simulink model "GTA_PCMFirmware"  (Simulink 7.8)
settings: Solver=FixedStepDiscrete  StartTime=0.0  StopTime=10.0  RelTol=1e-3
PreLoadFcn:
  | try, eval([bdroot '_setup']); catch, eval('model_setup', ''); end
InitFcn:
  | try, eval([bdroot '_setup']); catch, eval('model_setup', ''); end
undefined symbols (not defined in the file): fndFwd, fndNeut, fndRev, FWDlockout, GCM, keySwIgn2, motohawk_build_version, motohawk_trunc_name, motohawk_vardec_path, REVlockout
libraries: MotoHawk_lib x313, simulink x47, GTA_Library x13
(part 2 of 7)

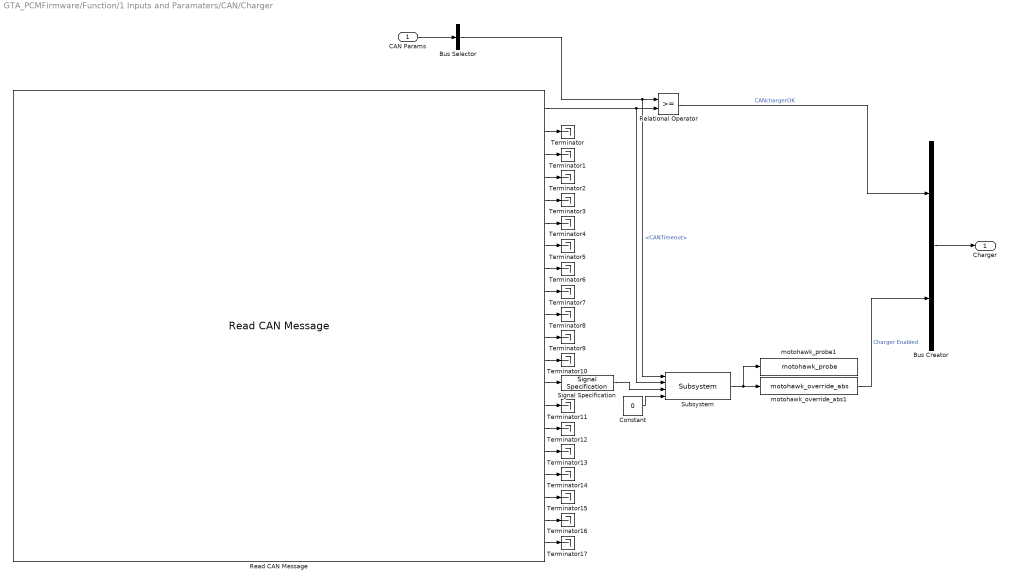
== system GTA_PCMFirmware/Function/1 Inputs and Paramaters/CAN/Charger ==
  CAN Params : Inport
  Bus Creator : BusCreator  Inputs=2
  Bus Selector : BusSelector  OutputSignals=CANTimeout
  Constant : Constant  Value=0  OutDataTypeStr=boolean
  Read CAN Message : MotoHawk_lib/CAN Blocks/Read CAN Message  nam='BMS_CAN'  bus=-2  msg=CANMSG_LHVcharger_Status  queue=1  slot=''  valid=off  stale=on  labelwires=off
  Relational Operator : RelationalOperator  OutDataTypeStr=boolean
  Signal Specification : SignalSpecification  OutDataTypeStr=boolean
  Subsystem : GTA_Library/Subsystem
  Terminator{,1..17} (18 alike) : Terminator
  motohawk_override_abs1 : MotoHawk_lib/Calibration & Probing Blocks/motohawk_override_abs  parent_name='ChargerEnabled'  parent_val=0  show_more=off  name_source=Use Parameter  parent_read_level=1  parent_override_level=1  view_as=Number  enum_struct={'Disabled', 'Enabled'}  use_help_units=off  parent_help=''  parent_units=''  use_min_max=off  parent_min=-inf  parent_max=inf  use_precision=off  parent_precision=''  parent_gain=1  parent_offset=0  parent_exp=1  use_mototune_group=off  parent_group=motohawk_vardec_path(gcb)
  motohawk_probe1 : MotoHawk_lib/Calibration & Probing Blocks/motohawk_probe  nam='ChargerEnabled'  show_more=off  name_source=Use Parameter  read_level=1  view_as=Number  enum_struct={'Disabled', 'Enabled'}  vector_style=Wide Row  use_help_units=off  help=''  units=''  use_header_enum=off  row_header_enum={}  col_header_enum={}  use_min_max=off  min_val=-inf  max_val=inf  use_precision=off  precision=''  gain=1  offset=0  exp=1  use_mototune_group=off  mototune_group=motohawk_vardec_path(gcb)
  Charger : Outport
  wires:
  CAN Params/1 -> Bus Selector/1
  Bus Selector/1 -> Relational Operator/1, Subsystem/1  "<CANTimeout>"
  Read CAN Message/1 -> Relational Operator/2, Subsystem/2
  Read CAN Message/2 -> Terminator/1
  Read CAN Message/3 -> Terminator1/1
  Read CAN Message/4 -> Terminator2/1
  Read CAN Message/5 -> Terminator3/1
  Read CAN Message/6 -> Terminator4/1
  Read CAN Message/7 -> Terminator5/1
  Read CAN Message/8 -> Terminator6/1
  Read CAN Message/9 -> Terminator7/1
  Read CAN Message/10 -> Terminator8/1
  Read CAN Message/11 -> Terminator9/1
  Read CAN Message/12 -> Terminator10/1
  Read CAN Message/14 -> Terminator11/1
  Read CAN Message/15 -> Terminator12/1
  Read CAN Message/16 -> Terminator13/1
  Read CAN Message/17 -> Terminator14/1
  Read CAN Message/18 -> Terminator15/1
  Read CAN Message/19 -> Terminator16/1
  Read CAN Message/20 -> Terminator17/1
  Read CAN Message/13 -> Signal Specification/1
  Constant/1 -> Subsystem/4
  Signal Specification/1 -> Subsystem/3
  Relational Operator/1 -> Bus Creator/1  "CANchargerOK"
  Bus Creator/1 -> Charger/1
  Subsystem/1 -> motohawk_override_abs1/1, motohawk_probe1/1
  motohawk_override_abs1/1 -> Bus Creator/2  "Charger Enabled"

== system GTA_PCMFirmware/Function/1 Inputs and Paramaters/Digital/Brake Switch ==
  Bus Creator : BusCreator  Inputs=1
  Data Type Conversion : DataTypeConversion  OutDataTypeStr=boolean
  Relay : Relay  OnSwitchValue=500  OffSwitchValue=400  OutDataTypeStr=uint8
  motohawk_ain : MotoHawk_lib/Analog I//O Blocks/motohawk_ain  res_name='BrakeSwitch'  text_resource=AN3M  code_resource=NONE  val_resource=-1  target=GCM-0563-048-0802  resource_enum_str=(None)=-1,LSD1=25,LSD2=26,ECUP=53,DRVP=54,XDRP=55,AN1M=56,AN2M=57,AN3M=58,AN4M=59,AN5M=60,AN6M=61,AN7M=62,AN8M=63,AN9M=64,AN10M=65,AN11M=66,AN12M=67,AN13M=68,AN14M=69,AN15M=70,AN16M=71,ESTOP=97,PWMADC=142  altref=5V Reference  typ=uint16  num_adc_bits=10  use_stat=off  use_vardec=off  nam='RTD1_MW'  read_level=1  write_level=1  group='System | I/O Pins | Inputs Config'
  motohawk_override_abs : MotoHawk_lib/Calibration & Probing Blocks/motohawk_override_abs  parent_name='BrakeSwitch'  parent_val=0  show_more=off  name_source=Use Parameter  parent_read_level=1  parent_override_level=1  view_as=Number  enum_struct={'Disabled', 'Enabled'}  use_help_units=off  parent_help=''  parent_units=''  use_min_max=off  parent_min=-inf  parent_max=inf  use_precision=off  parent_precision=''  parent_gain=1  parent_offset=0  parent_exp=1  use_mototune_group=off  parent_group=motohawk_vardec_path(gcb)
  motohawk_probe : MotoHawk_lib/Calibration & Probing Blocks/motohawk_probe  nam='BrakeSwitch'  show_more=off  name_source=Use Parameter  read_level=1  view_as=Number  enum_struct={'Disabled', 'Enabled'}  vector_style=Wide Row  use_help_units=off  help=''  units=''  use_header_enum=off  row_header_enum={}  col_header_enum={}  use_min_max=off  min_val=-inf  max_val=inf  use_precision=off  precision=''  gain=1  offset=0  exp=1  use_mototune_group=off  mototune_group=motohawk_vardec_path(gcb)
  BrakeSwitch : Outport
  wires:
  motohawk_ain/1 -> Relay/1
  Relay/1 -> Data Type Conversion/1
  Data Type Conversion/1 -> motohawk_override_abs/1, motohawk_probe/1
  motohawk_override_abs/1 -> Bus Creator/1  "BrakeSw"
  Bus Creator/1 -> BrakeSwitch/1

== system GTA_PCMFirmware/Function/1 Inputs and Paramaters/Digital/Charger ==
  Bus Creator : BusCreator  Inputs=1
  Data Type Conversion : DataTypeConversion  OutDataTypeStr=boolean
  Relay : Relay  OnSwitchValue=150  OffSwitchValue=100  OutDataTypeStr=uint8
  motohawk_ain : MotoHawk_lib/Analog I//O Blocks/motohawk_ain  res_name='ACPresent'  text_resource=AN13M  code_resource=NONE  val_resource=-1  target=GCM-0563-048-0802  resource_enum_str=(None)=-1,LSD1=25,LSD2=26,ECUP=53,DRVP=54,XDRP=55,AN1M=56,AN2M=57,AN3M=58,AN4M=59,AN5M=60,AN6M=61,AN7M=62,AN8M=63,AN9M=64,AN10M=65,AN11M=66,AN12M=67,AN13M=68,AN14M=69,AN15M=70,AN16M=71,ESTOP=97,PWMADC=142  altref=5V Reference  typ=uint16  num_adc_bits=10  use_stat=off  use_vardec=off  nam='RTD1_MW'  read_level=1  write_level=1  group='System | I/O Pins | Inputs Config'
  motohawk_override_abs : MotoHawk_lib/Calibration & Probing Blocks/motohawk_override_abs  parent_name='AC_Present'  parent_val=0  show_more=off  name_source=Use Parameter  parent_read_level=1  parent_override_level=1  view_as=Number  enum_struct={'Disabled', 'Enabled'}  use_help_units=off  parent_help=''  parent_units=''  use_min_max=off  parent_min=-inf  parent_max=inf  use_precision=off  parent_precision=''  parent_gain=1  parent_offset=0  parent_exp=1  use_mototune_group=off  parent_group=motohawk_vardec_path(gcb)
  motohawk_probe : MotoHawk_lib/Calibration & Probing Blocks/motohawk_probe  nam='AC_Present'  show_more=off  name_source=Use Parameter  read_level=1  view_as=Number  enum_struct={'Disabled', 'Enabled'}  vector_style=Wide Row  use_help_units=off  help=''  units=''  use_header_enum=off  row_header_enum={}  col_header_enum={}  use_min_max=off  min_val=-inf  max_val=inf  use_precision=off  precision=''  gain=1  offset=0  exp=1  use_mototune_group=off  mototune_group=motohawk_vardec_path(gcb)
  Charger : Outport
  wires:
  motohawk_ain/1 -> Relay/1
  Relay/1 -> Data Type Conversion/1
  Bus Creator/1 -> Charger/1
  Data Type Conversion/1 -> motohawk_override_abs/1, motohawk_probe/1
  motohawk_override_abs/1 -> Bus Creator/1  "acPresent"

== system GTA_PCMFirmware/Function/1 Inputs and Paramaters/Digital/EStop ==
  Bus Creator : BusCreator  Inputs=1
  Data Type Conversion : DataTypeConversion  OutDataTypeStr=boolean
  Relay : Relay  OnSwitchValue=500  OffSwitchValue=400  OutDataTypeStr=uint8
  motohawk_ain : MotoHawk_lib/Analog I//O Blocks/motohawk_ain  res_name='EStopSwitch'  text_resource=AN12M  code_resource=NONE  val_resource=-1  target=GCM-0563-048-0802  resource_enum_str=(None)=-1,LSD1=25,LSD2=26,ECUP=53,DRVP=54,XDRP=55,AN1M=56,AN2M=57,AN3M=58,AN4M=59,AN5M=60,AN6M=61,AN7M=62,AN8M=63,AN9M=64,AN10M=65,AN11M=66,AN12M=67,AN13M=68,AN14M=69,AN15M=70,AN16M=71,ESTOP=97,PWMADC=142  altref=5V Reference  typ=uint16  num_adc_bits=10  use_stat=off  use_vardec=off  nam='RTD1_MW'  read_level=1  write_level=1  group='System | I/O Pins | Inputs Config'
  motohawk_override_abs : MotoHawk_lib/Calibration & Probing Blocks/motohawk_override_abs  parent_name='EStop'  parent_val=0  show_more=off  name_source=Use Parameter  parent_read_level=1  parent_override_level=1  view_as=Number  enum_struct={'Disabled', 'Enabled'}  use_help_units=off  parent_help=''  parent_units=''  use_min_max=off  parent_min=-inf  parent_max=inf  use_precision=off  parent_precision=''  parent_gain=1  parent_offset=0  parent_exp=1  use_mototune_group=off  parent_group=motohawk_vardec_path(gcb)
  motohawk_probe : MotoHawk_lib/Calibration & Probing Blocks/motohawk_probe  nam='EStop'  show_more=off  name_source=Use Parameter  read_level=1  view_as=Number  enum_struct={'Disabled', 'Enabled'}  vector_style=Wide Row  use_help_units=off  help=''  units=''  use_header_enum=off  row_header_enum={}  col_header_enum={}  use_min_max=off  min_val=-inf  max_val=inf  use_precision=off  precision=''  gain=1  offset=0  exp=1  use_mototune_group=off  mototune_group=motohawk_vardec_path(gcb)
  Estop : Outport
  wires:
  motohawk_ain/1 -> Relay/1
  Relay/1 -> Data Type Conversion/1
  Data Type Conversion/1 -> motohawk_override_abs/1, motohawk_probe/1
  motohawk_override_abs/1 -> Bus Creator/1  "EStop"
  Bus Creator/1 -> Estop/1

== system GTA_PCMFirmware/Function/1 Inputs and Paramaters/Digital/Key Switch ==
  note: Ign1 += 1
      | Ign2 += 2
      | Crank += 4
  Add : Sum  Inputs=|++  AccumDataTypeStr=uint8
  Bus Creator : BusCreator  Inputs=2
  Bus Creator1 : BusCreator  Inputs=2
  Data Type Conversion : DataTypeConversion  OutDataTypeStr=boolean
  Data Type Conversion1 : DataTypeConversion  OutDataTypeStr=boolean
  Relay : Relay  OnSwitchValue=150  OffSwitchValue=100  OnOutputValue=keySwIgn2  OutDataTypeStr=uint8
  Relay1 : Relay  OnSwitchValue=150  OffSwitchValue=100  OnOutputValue=keySwCrank  OutDataTypeStr=uint8
  motohawk_ain1 : MotoHawk_lib/Analog I//O Blocks/motohawk_ain  res_name='keySwIgn2'  text_resource=AN14M  code_resource=NONE  val_resource=-1  target=GCM-0563-048-0802  resource_enum_str=(None)=-1,LSD1=25,LSD2=26,ECUP=53,DRVP=54,XDRP=55,AN1M=56,AN2M=57,AN3M=58,AN4M=59,AN5M=60,AN6M=61,AN7M=62,AN8M=63,AN9M=64,AN10M=65,AN11M=66,AN12M=67,AN13M=68,AN14M=69,AN15M=70,AN16M=71,ESTOP=97,PWMADC=142  altref=5V Reference  typ=uint16  num_adc_bits=10  use_stat=off  use_vardec=off  nam='RTD1_MW'  read_level=1  write_level=1  group='System | I/O Pins | Inputs Config'
  motohawk_ain2 : MotoHawk_lib/Analog I//O Blocks/motohawk_ain  res_name='keySwCrank'  text_resource=AN16M  code_resource=NONE  val_resource=-1  target=GCM-0563-048-0802  resource_enum_str=(None)=-1,LSD1=25,LSD2=26,ECUP=53,DRVP=54,XDRP=55,AN1M=56,AN2M=57,AN3M=58,AN4M=59,AN5M=60,AN6M=61,AN7M=62,AN8M=63,AN9M=64,AN10M=65,AN11M=66,AN12M=67,AN13M=68,AN14M=69,AN15M=70,AN16M=71,ESTOP=97,PWMADC=142  altref=5V Reference  typ=uint16  num_adc_bits=10  use_stat=off  use_vardec=off  nam='RTD1_MW'  read_level=1  write_level=1  group='System | I/O Pins | Inputs Config'
  motohawk_override_abs : MotoHawk_lib/Calibration & Probing Blocks/motohawk_override_abs  parent_name='KeySw'  parent_val=0  show_more=off  name_source=Use Parameter  parent_read_level=1  parent_override_level=1  view_as=Number  enum_struct={'Disabled', 'Enabled'}  use_help_units=off  parent_help=''  parent_units=''  use_min_max=off  parent_min=-inf  parent_max=inf  use_precision=off  parent_precision=''  parent_gain=1  parent_offset=0  parent_exp=1  use_mototune_group=off  parent_group=motohawk_vardec_path(gcb)
  motohawk_probe : MotoHawk_lib/Calibration & Probing Blocks/motohawk_probe  nam='KeySw'  show_more=off  name_source=Use Parameter  read_level=1  view_as=Number  enum_struct={'Disabled', 'Enabled'}  vector_style=Wide Row  use_help_units=off  help=''  units=''  use_header_enum=off  row_header_enum={}  col_header_enum={}  use_min_max=off  min_val=-inf  max_val=inf  use_precision=off  precision=''  gain=1  offset=0  exp=1  use_mototune_group=off  mototune_group=motohawk_vardec_path(gcb)
  KeySw : Outport
  wires:
  motohawk_ain1/1 -> Relay/1
  motohawk_ain2/1 -> Relay1/1
  Relay/1 -> Add/1, Data Type Conversion/1
  Relay1/1 -> Add/2, Data Type Conversion1/1
  Add/1 -> motohawk_override_abs/1, motohawk_probe/1
  motohawk_override_abs/1 -> Bus Creator1/1  "KeySw"
  Data Type Conversion/1 -> Bus Creator/1  "dbgIGN2"
  Data Type Conversion1/1 -> Bus Creator/2  "dbgCrank"
  Bus Creator1/1 -> KeySw/1
  Bus Creator/1 -> Bus Creator1/2  "dbgKeySW"

== system GTA_PCMFirmware/Function/1 Inputs and Paramaters/Digital/Rear Defrost Switch ==
  Bus Creator : BusCreator  Inputs=1
  Data Type Conversion : DataTypeConversion  OutDataTypeStr=boolean
  Relay : Relay  OnSwitchValue=500  OffSwitchValue=400  OnOutputValue=0  OffOutputValue=1  OutDataTypeStr=uint8
  motohawk_ain : MotoHawk_lib/Analog I//O Blocks/motohawk_ain  res_name='RearDefrostSwitch'  text_resource=AN11M  code_resource=NONE  val_resource=-1  target=GCM-0563-048-0802  resource_enum_str=(None)=-1,LSD1=25,LSD2=26,ECUP=53,DRVP=54,XDRP=55,AN1M=56,AN2M=57,AN3M=58,AN4M=59,AN5M=60,AN6M=61,AN7M=62,AN8M=63,AN9M=64,AN10M=65,AN11M=66,AN12M=67,AN13M=68,AN14M=69,AN15M=70,AN16M=71,ESTOP=97,PWMADC=142  altref=5V Reference  typ=uint16  num_adc_bits=10  use_stat=off  use_vardec=off  nam='RTD1_MW'  read_level=1  write_level=1  group='System | I/O Pins | Inputs Config'
  motohawk_override_abs : MotoHawk_lib/Calibration & Probing Blocks/motohawk_override_abs  parent_name='DefrostSW'  parent_val=0  show_more=off  name_source=Use Parameter  parent_read_level=1  parent_override_level=1  view_as=Number  enum_struct={'Disabled', 'Enabled'}  use_help_units=off  parent_help=''  parent_units=''  use_min_max=off  parent_min=-inf  parent_max=inf  use_precision=off  parent_precision=''  parent_gain=1  parent_offset=0  parent_exp=1  use_mototune_group=off  parent_group=motohawk_vardec_path(gcb)
  motohawk_probe : MotoHawk_lib/Calibration & Probing Blocks/motohawk_probe  nam='DefrostSW'  show_more=off  name_source=Use Parameter  read_level=1  view_as=Number  enum_struct={'Disabled', 'Enabled'}  vector_style=Wide Row  use_help_units=off  help=''  units=''  use_header_enum=off  row_header_enum={}  col_header_enum={}  use_min_max=off  min_val=-inf  max_val=inf  use_precision=off  precision=''  gain=1  offset=0  exp=1  use_mototune_group=off  mototune_group=motohawk_vardec_path(gcb)
  DefrostSW : Outport
  wires:
  motohawk_ain/1 -> Relay/1
  Relay/1 -> Data Type Conversion/1
  Data Type Conversion/1 -> motohawk_override_abs/1, motohawk_probe/1
  motohawk_override_abs/1 -> Bus Creator/1  "DefrostSW"
  Bus Creator/1 -> DefrostSW/1

== system GTA_PCMFirmware/Function/1 Inputs and Paramaters/Digital/Shifter ==
  note: Neutral = 0, Reverse = 1, Forward = 2
  Bus Creator : BusCreator  Inputs=2
  Combinatorial  Logic : CombinatorialLogic  TruthTable=[0; 0; 0; 0; 0; 0; 0; 0; 0; 2; 0; 0; 1; 0; 0; 0;]
  Combinatorial  Logic1 : CombinatorialLogic  TruthTable=[4; 4; 4; 4; 4; 0; 4; 4; 4; 2; 4; 4; 1; 4; 4; 4;]
  Constant : Constant  Value=0  OutDataTypeStr=uint16
  Data Type Conversion : DataTypeConversion  OutDataTypeStr=boolean
  Data Type Conversion1 : DataTypeConversion  OutDataTypeStr=uint8
  Mux : Mux
  Relay{,1..3} (4 alike) : Relay  OnSwitchValue=150  OffSwitchValue=100  OutDataTypeStr=uint8
  ShifterDebug : Subsystem
  motohawk_ain : MotoHawk_lib/Analog I//O Blocks/motohawk_ain  res_name='SHIFTER_GLS0'  text_resource=AN5M  code_resource=NONE  val_resource=-1  target=GCM-0563-048-0802  resource_enum_str=(None)=-1,LSD1=25,LSD2=26,ECUP=53,DRVP=54,XDRP=55,AN1M=56,AN2M=57,AN3M=58,AN4M=59,AN5M=60,AN6M=61,AN7M=62,AN8M=63,AN9M=64,AN10M=65,AN11M=66,AN12M=67,AN13M=68,AN14M=69,AN15M=70,AN16M=71,ESTOP=97,PWMADC=142  altref=5V Reference  typ=uint16  num_adc_bits=10  use_stat=off  use_vardec=off  nam='RTD1_MW'  read_level=1  write_level=1  group='System | I/O Pins | Inputs Config'
  motohawk_ain1 : MotoHawk_lib/Analog I//O Blocks/motohawk_ain  res_name='SHIFTER_GLS1'  text_resource=AN6M  code_resource=NONE  val_resource=-1  target=GCM-0563-048-0802  resource_enum_str=(None)=-1,LSD1=25,LSD2=26,ECUP=53,DRVP=54,XDRP=55,AN1M=56,AN2M=57,AN3M=58,AN4M=59,AN5M=60,AN6M=61,AN7M=62,AN8M=63,AN9M=64,AN10M=65,AN11M=66,AN12M=67,AN13M=68,AN14M=69,AN15M=70,AN16M=71,ESTOP=97,PWMADC=142  altref=5V Reference  typ=uint16  num_adc_bits=10  use_stat=off  use_vardec=off  nam='RTD1_MW'  read_level=1  write_level=1  group='System | I/O Pins | Inputs Config'
  motohawk_ain2 : MotoHawk_lib/Analog I//O Blocks/motohawk_ain  res_name='SHIFTER_GLS3'  text_resource=AN7M  code_resource=NONE  val_resource=-1  target=GCM-0563-048-0802  resource_enum_str=(None)=-1,LSD1=25,LSD2=26,ECUP=53,DRVP=54,XDRP=55,AN1M=56,AN2M=57,AN3M=58,AN4M=59,AN5M=60,AN6M=61,AN7M=62,AN8M=63,AN9M=64,AN10M=65,AN11M=66,AN12M=67,AN13M=68,AN14M=69,AN15M=70,AN16M=71,ESTOP=97,PWMADC=142  altref=5V Reference  typ=uint16  num_adc_bits=10  use_stat=off  use_vardec=off  nam='RTD1_MW'  read_level=1  write_level=1  group='System | I/O Pins | Inputs Config'
  motohawk_override_abs : MotoHawk_lib/Calibration & Probing Blocks/motohawk_override_abs  parent_name='Shifter'  parent_val=0  show_more=off  name_source=Use Parameter  parent_read_level=1  parent_override_level=1  view_as=Number  enum_struct={'Disabled', 'Enabled'}  use_help_units=off  parent_help=''  parent_units=''  use_min_max=off  parent_min=-inf  parent_max=inf  use_precision=off  parent_precision=''  parent_gain=1  parent_offset=0  parent_exp=1  use_mototune_group=off  parent_group=motohawk_vardec_path(gcb)
  motohawk_probe : MotoHawk_lib/Calibration & Probing Blocks/motohawk_probe  nam='Shifter'  show_more=off  name_source=Use Parameter  read_level=1  view_as=Number  enum_struct={'Disabled', 'Enabled'}  vector_style=Wide Row  use_help_units=off  help=''  units=''  use_header_enum=off  row_header_enum={}  col_header_enum={}  use_min_max=off  min_val=-inf  max_val=inf  use_precision=off  precision=''  gain=1  offset=0  exp=1  use_mototune_group=off  mototune_group=motohawk_vardec_path(gcb)
  Shifter : Outport
  wires:
  Relay/1 -> Mux/1
  Relay1/1 -> Mux/2
  Relay2/1 -> Mux/3
  Relay3/1 -> Mux/4
  Constant/1 -> Relay2/1
  motohawk_ain1/1 -> Relay1/1
  motohawk_ain/1 -> Relay/1
  motohawk_ain2/1 -> Relay3/1
  Mux/1 -> Data Type Conversion/1
  Data Type Conversion/1 -> Combinatorial  Logic/1, Combinatorial  Logic1/1
  Combinatorial  Logic/1 -> motohawk_override_abs/1, motohawk_probe/1
  motohawk_override_abs/1 -> Data Type Conversion1/1  "Shifter"
  Bus Creator/1 -> Shifter/1
  Combinatorial  Logic1/1 -> ShifterDebug/1(Shift_out)
  ShifterDebug/1(dbgShifter) -> Bus Creator/2  "dbgShifter"
  Data Type Conversion1/1 -> Bus Creator/1  "ShifterPos"

== system GTA_PCMFirmware/Function/1 Inputs and Paramaters/Digital/Wiper Enable ==
  Bus Creator : BusCreator  Inputs=1
  motohawk_din : MotoHawk_lib/Digital I//O Blocks/motohawk_din  resource_name='Wipen_Enable'  text_resource=DG1M  code_resource=NONE  val_resource=-1  target=GCM-0563-048-0802  resource_enum_str=(None)=-1,AN1M=56,AN2M=57,AN3M=58,AN4M=59,AN5M=60,AN6M=61,AN7M=62,AN8M=63,AN9M=64,AN10M=65,AN11M=66,AN12M=67,AN13M=68,AN14M=69,AN15M=70,AN16M=71,DG1M=93,DG2M=94,DG3M=95,DG4M=96,ESTOP=97,DG5M=102,DG6M=103  pullup=None  use_stat=off  use_vardec=off  nam='DIN'  read_level=1  write_level=1  group='System | I/O Pins | Inputs Config'
  motohawk_override_abs : MotoHawk_lib/Calibration & Probing Blocks/motohawk_override_abs  parent_name='WiperSw'  parent_val=0  show_more=off  name_source=Use Parameter  parent_read_level=1  parent_override_level=1  view_as=Number  enum_struct={'Disabled', 'Enabled'}  use_help_units=off  parent_help=''  parent_units=''  use_min_max=off  parent_min=-inf  parent_max=inf  use_precision=off  parent_precision=''  parent_gain=1  parent_offset=0  parent_exp=1  use_mototune_group=off  parent_group=motohawk_vardec_path(gcb)
  motohawk_probe : MotoHawk_lib/Calibration & Probing Blocks/motohawk_probe  nam='WiperSw'  show_more=off  name_source=Use Parameter  read_level=1  view_as=Number  enum_struct={'Disabled', 'Enabled'}  vector_style=Wide Row  use_help_units=off  help=''  units=''  use_header_enum=off  row_header_enum={}  col_header_enum={}  use_min_max=off  min_val=-inf  max_val=inf  use_precision=off  precision=''  gain=1  offset=0  exp=1  use_mototune_group=off  mototune_group=motohawk_vardec_path(gcb)
  WiperSw : Outport
  wires:
  motohawk_din/1 -> motohawk_override_abs/1, motohawk_probe/1
  motohawk_override_abs/1 -> Bus Creator/1  "WiperSw"
  Bus Creator/1 -> WiperSw/1

== system GTA_PCMFirmware/Function/1 Inputs and Paramaters/Limits/Li15kWh ==
  Mux : Mux  Inputs=13
  motohawk_calibration : MotoHawk_lib/Calibration & Probing Blocks/motohawk_calibration  nam='Li15MaxCellVoltage'  val=Li15MaxCellVoltage  storage=Calibration  show_more=off  name_source=Use Parameter  data_type=Inherit from 'Default Value'  read_level=1  write_level=1  ovr_cals=on  view_as=Number  enum_struct={'Disabled', 'Enabled'}  vector_style=Wide Row  use_help_units=off  help=''  units=''  use_header_enum=off  row_header_enum={}  col_header_enum={}  use_min_max=off  min_val=-inf  max_val=inf  use_precision=off  precision=''  gain=1  offset=0  exp=1  use_mototune_group=off  mototune_group=motohawk_vardec_path(gcb)
  motohawk_calibration1 : MotoHawk_lib/Calibration & Probing Blocks/motohawk_calibration  nam='Li15MinCellVoltage'  val=Li15MinCellVoltage  storage=Calibration  show_more=off  name_source=Use Parameter  data_type=Inherit from 'Default Value'  read_level=1  write_level=1  ovr_cals=on  view_as=Number  enum_struct={'Disabled', 'Enabled'}  vector_style=Wide Row  use_help_units=off  help=''  units=''  use_header_enum=off  row_header_enum={}  col_header_enum={}  use_min_max=off  min_val=-inf  max_val=inf  use_precision=off  precision=''  gain=1  offset=0  exp=1  use_mototune_group=off  mototune_group=motohawk_vardec_path(gcb)
  motohawk_calibration10 : MotoHawk_lib/Calibration & Probing Blocks/motohawk_calibration  nam='Li15MotorCurrentScalar'  val=Li15MotorCurrentScalar  storage=Calibration  show_more=off  name_source=Use Parameter  data_type=Inherit from 'Default Value'  read_level=1  write_level=1  ovr_cals=on  view_as=Number  enum_struct={'Disabled', 'Enabled'}  vector_style=Wide Row  use_help_units=off  help=''  units=''  use_header_enum=off  row_header_enum={}  col_header_enum={}  use_min_max=off  min_val=-inf  max_val=inf  use_precision=off  precision=''  gain=1  offset=0  exp=1  use_mototune_group=off  mototune_group=motohawk_vardec_path(gcb)
  motohawk_calibration11 : MotoHawk_lib/Calibration & Probing Blocks/motohawk_calibration  nam='Li15MotorRegenScalar'  val=Li15MotorRegenScalar  storage=Calibration  show_more=off  name_source=Use Parameter  data_type=Inherit from 'Default Value'  read_level=1  write_level=1  ovr_cals=on  view_as=Number  enum_struct={'Disabled', 'Enabled'}  vector_style=Wide Row  use_help_units=off  help=''  units=''  use_header_enum=off  row_header_enum={}  col_header_enum={}  use_min_max=off  min_val=-inf  max_val=inf  use_precision=off  precision=''  gain=1  offset=0  exp=1  use_mototune_group=off  mototune_group=motohawk_vardec_path(gcb)
  motohawk_calibration12 : MotoHawk_lib/Calibration & Probing Blocks/motohawk_calibration  nam='Li15MaxRegenVoltage'  val=Li15MaxRegenVoltage  storage=Calibration  show_more=off  name_source=Use Parameter  data_type=Inherit from 'Default Value'  read_level=1  write_level=1  ovr_cals=on  view_as=Number  enum_struct={'Disabled', 'Enabled'}  vector_style=Wide Row  use_help_units=off  help=''  units=''  use_header_enum=off  row_header_enum={}  col_header_enum={}  use_min_max=off  min_val=-inf  max_val=inf  use_precision=off  precision=''  gain=1  offset=0  exp=1  use_mototune_group=off  mototune_group=motohawk_vardec_path(gcb)
  motohawk_calibration2 : MotoHawk_lib/Calibration & Probing Blocks/motohawk_calibration  nam='Li15CurrentLimit'  val=Li15CurrentLimit  storage=Calibration  show_more=off  name_source=Use Parameter  data_type=Inherit from 'Default Value'  read_level=1  write_level=1  ovr_cals=on  view_as=Number  enum_struct={'Disabled', 'Enabled'}  vector_style=Wide Row  use_help_units=off  help=''  units=''  use_header_enum=off  row_header_enum={}  col_header_enum={}  use_min_max=off  min_val=-inf  max_val=inf  use_precision=off  precision=''  gain=1  offset=0  exp=1  use_mototune_group=off  mototune_group=motohawk_vardec_path(gcb)
  motohawk_calibration3 : MotoHawk_lib/Calibration & Probing Blocks/motohawk_calibration  nam='Li15RegenLimit'  val=Li15RegenLimit  storage=Calibration  show_more=off  name_source=Use Parameter  data_type=Inherit from 'Default Value'  read_level=1  write_level=1  ovr_cals=on  view_as=Number  enum_struct={'Disabled', 'Enabled'}  vector_style=Wide Row  use_help_units=off  help=''  units=''  use_header_enum=off  row_header_enum={}  col_header_enum={}  use_min_max=off  min_val=-inf  max_val=inf  use_precision=off  precision=''  gain=1  offset=0  exp=1  use_mototune_group=off  mototune_group=motohawk_vardec_path(gcb)
  motohawk_calibration4 : MotoHawk_lib/Calibration & Probing Blocks/motohawk_calibration  nam='Li15MaxChargeTemp'  val=Li15MaxChargeTemp  storage=Calibration  show_more=off  name_source=Use Parameter  data_type=Inherit from 'Default Value'  read_level=1  write_level=1  ovr_cals=on  view_as=Number  enum_struct={'Disabled', 'Enabled'}  vector_style=Wide Row  use_help_units=off  help=''  units=''  use_header_enum=off  row_header_enum={}  col_header_enum={}  use_min_max=off  min_val=-inf  max_val=inf  use_precision=off  precision=''  gain=1  offset=0  exp=1  use_mototune_group=off  mototune_group=motohawk_vardec_path(gcb)
  motohawk_calibration5 : MotoHawk_lib/Calibration & Probing Blocks/motohawk_calibration  nam='Li15MinChargeTemp'  val=Li15MinChargeTemp  storage=Calibration  show_more=off  name_source=Use Parameter  data_type=Inherit from 'Default Value'  read_level=1  write_level=1  ovr_cals=on  view_as=Number  enum_struct={'Disabled', 'Enabled'}  vector_style=Wide Row  use_help_units=off  help=''  units=''  use_header_enum=off  row_header_enum={}  col_header_enum={}  use_min_max=off  min_val=-inf  max_val=inf  use_precision=off  precision=''  gain=1  offset=0  exp=1  use_mototune_group=off  mototune_group=motohawk_vardec_path(gcb)
  motohawk_calibration6 : MotoHawk_lib/Calibration & Probing Blocks/motohawk_calibration  nam='Li15MaxDischargeTemp'  val=Li15MaxDischargeTemp  storage=Calibration  show_more=off  name_source=Use Parameter  data_type=Inherit from 'Default Value'  read_level=1  write_level=1  ovr_cals=on  view_as=Number  enum_struct={'Disabled', 'Enabled'}  vector_style=Wide Row  use_help_units=off  help=''  units=''  use_header_enum=off  row_header_enum={}  col_header_enum={}  use_min_max=off  min_val=-inf  max_val=inf  use_precision=off  precision=''  gain=1  offset=0  exp=1  use_mototune_group=off  mototune_group=motohawk_vardec_path(gcb)
  motohawk_calibration7 : MotoHawk_lib/Calibration & Probing Blocks/motohawk_calibration  nam='Li15MinDischargeTemp'  val=Li15MinDischargeTemp  storage=Calibration  show_more=off  name_source=Use Parameter  data_type=Inherit from 'Default Value'  read_level=1  write_level=1  ovr_cals=on  view_as=Number  enum_struct={'Disabled', 'Enabled'}  vector_style=Wide Row  use_help_units=off  help=''  units=''  use_header_enum=off  row_header_enum={}  col_header_enum={}  use_min_max=off  min_val=-inf  max_val=inf  use_precision=off  precision=''  gain=1  offset=0  exp=1  use_mototune_group=off  mototune_group=motohawk_vardec_path(gcb)
  motohawk_calibration8 : MotoHawk_lib/Calibration & Probing Blocks/motohawk_calibration  nam='Li15MaxPackVoltage'  val=Li15MaxPackVoltage  storage=Calibration  show_more=off  name_source=Use Parameter  data_type=Inherit from 'Default Value'  read_level=1  write_level=1  ovr_cals=on  view_as=Number  enum_struct={'Disabled', 'Enabled'}  vector_style=Wide Row  use_help_units=off  help=''  units=''  use_header_enum=off  row_header_enum={}  col_header_enum={}  use_min_max=off  min_val=-inf  max_val=inf  use_precision=off  precision=''  gain=1  offset=0  exp=1  use_mototune_group=off  mototune_group=motohawk_vardec_path(gcb)
  motohawk_calibration9 : MotoHawk_lib/Calibration & Probing Blocks/motohawk_calibration  nam='Li15MinPackVoltage'  val=Li15MinPackVoltage  storage=Calibration  show_more=off  name_source=Use Parameter  data_type=Inherit from 'Default Value'  read_level=1  write_level=1  ovr_cals=on  view_as=Number  enum_struct={'Disabled', 'Enabled'}  vector_style=Wide Row  use_help_units=off  help=''  units=''  use_header_enum=off  row_header_enum={}  col_header_enum={}  use_min_max=off  min_val=-inf  max_val=inf  use_precision=off  precision=''  gain=1  offset=0  exp=1  use_mototune_group=off  mototune_group=motohawk_vardec_path(gcb)
  Li15Pack : Outport
  wires:
  motohawk_calibration12/1 -> Mux/13  "MaxRegenVoltage"
  motohawk_calibration11/1 -> Mux/12  "MotorRegenScalar"
  motohawk_calibration10/1 -> Mux/11  "MotorCurrentScalar"
  motohawk_calibration9/1 -> Mux/10  "MinPackVoltage"
  motohawk_calibration8/1 -> Mux/9  "MaxPackVoltage"
  motohawk_calibration7/1 -> Mux/8  "MinDischargeTemp"
  motohawk_calibration6/1 -> Mux/7  "MaxDischargeTemp"
  motohawk_calibration5/1 -> Mux/6  "MinChargeTemp"
  motohawk_calibration4/1 -> Mux/5  "MaxChargeTemp"
  motohawk_calibration3/1 -> Mux/4  "RegenLimit"
  motohawk_calibration2/1 -> Mux/3  "CurrentLimit"
  motohawk_calibration1/1 -> Mux/2  "MinCellVoltage"
  motohawk_calibration/1 -> Mux/1  "MaxCellVoltage"
  Mux/1 -> Li15Pack/1

== system GTA_PCMFirmware/Function/1 Inputs and Paramaters/Limits/Li23kWh ==
  Mux : Mux  Inputs=13
  motohawk_calibration : MotoHawk_lib/Calibration & Probing Blocks/motohawk_calibration  nam='Li23MaxCellVoltage'  val=Li23MaxCellVoltage  storage=Calibration  show_more=off  name_source=Use Parameter  data_type=Inherit from 'Default Value'  read_level=1  write_level=1  ovr_cals=on  view_as=Number  enum_struct={'Disabled', 'Enabled'}  vector_style=Wide Row  use_help_units=off  help=''  units=''  use_header_enum=off  row_header_enum={}  col_header_enum={}  use_min_max=off  min_val=-inf  max_val=inf  use_precision=off  precision=''  gain=1  offset=0  exp=1  use_mototune_group=off  mototune_group=motohawk_vardec_path(gcb)
  motohawk_calibration1 : MotoHawk_lib/Calibration & Probing Blocks/motohawk_calibration  nam='Li23MinCellVoltage'  val=Li23MinCellVoltage  storage=Calibration  show_more=off  name_source=Use Parameter  data_type=Inherit from 'Default Value'  read_level=1  write_level=1  ovr_cals=on  view_as=Number  enum_struct={'Disabled', 'Enabled'}  vector_style=Wide Row  use_help_units=off  help=''  units=''  use_header_enum=off  row_header_enum={}  col_header_enum={}  use_min_max=off  min_val=-inf  max_val=inf  use_precision=off  precision=''  gain=1  offset=0  exp=1  use_mototune_group=off  mototune_group=motohawk_vardec_path(gcb)
  motohawk_calibration10 : MotoHawk_lib/Calibration & Probing Blocks/motohawk_calibration  nam='Li23MotorCurrentScalar'  val=Li23MotorCurrentScalar  storage=Calibration  show_more=off  name_source=Use Parameter  data_type=Inherit from 'Default Value'  read_level=1  write_level=1  ovr_cals=on  view_as=Number  enum_struct={'Disabled', 'Enabled'}  vector_style=Wide Row  use_help_units=off  help=''  units=''  use_header_enum=off  row_header_enum={}  col_header_enum={}  use_min_max=off  min_val=-inf  max_val=inf  use_precision=off  precision=''  gain=1  offset=0  exp=1  use_mototune_group=off  mototune_group=motohawk_vardec_path(gcb)
  motohawk_calibration11 : MotoHawk_lib/Calibration & Probing Blocks/motohawk_calibration  nam='Li23MotorRegenScalar'  val=Li23MotorRegenScalar  storage=Calibration  show_more=off  name_source=Use Parameter  data_type=Inherit from 'Default Value'  read_level=1  write_level=1  ovr_cals=on  view_as=Number  enum_struct={'Disabled', 'Enabled'}  vector_style=Wide Row  use_help_units=off  help=''  units=''  use_header_enum=off  row_header_enum={}  col_header_enum={}  use_min_max=off  min_val=-inf  max_val=inf  use_precision=off  precision=''  gain=1  offset=0  exp=1  use_mototune_group=off  mototune_group=motohawk_vardec_path(gcb)
  motohawk_calibration12 : MotoHawk_lib/Calibration & Probing Blocks/motohawk_calibration  nam='Li23MaxRegenVoltage'  val=Li23MaxRegenVoltage  storage=Calibration  show_more=off  name_source=Use Parameter  data_type=Inherit from 'Default Value'  read_level=1  write_level=1  ovr_cals=on  view_as=Number  enum_struct={'Disabled', 'Enabled'}  vector_style=Wide Row  use_help_units=off  help=''  units=''  use_header_enum=off  row_header_enum={}  col_header_enum={}  use_min_max=off  min_val=-inf  max_val=inf  use_precision=off  precision=''  gain=1  offset=0  exp=1  use_mototune_group=off  mototune_group=motohawk_vardec_path(gcb)
  motohawk_calibration2 : MotoHawk_lib/Calibration & Probing Blocks/motohawk_calibration  nam='Li23CurrentLimit'  val=Li23CurrentLimit  storage=Calibration  show_more=off  name_source=Use Parameter  data_type=Inherit from 'Default Value'  read_level=1  write_level=1  ovr_cals=on  view_as=Number  enum_struct={'Disabled', 'Enabled'}  vector_style=Wide Row  use_help_units=off  help=''  units=''  use_header_enum=off  row_header_enum={}  col_header_enum={}  use_min_max=off  min_val=-inf  max_val=inf  use_precision=off  precision=''  gain=1  offset=0  exp=1  use_mototune_group=off  mototune_group=motohawk_vardec_path(gcb)
  motohawk_calibration3 : MotoHawk_lib/Calibration & Probing Blocks/motohawk_calibration  nam='Li23RegenLimit'  val=Li23RegenLimit  storage=Calibration  show_more=off  name_source=Use Parameter  data_type=Inherit from 'Default Value'  read_level=1  write_level=1  ovr_cals=on  view_as=Number  enum_struct={'Disabled', 'Enabled'}  vector_style=Wide Row  use_help_units=off  help=''  units=''  use_header_enum=off  row_header_enum={}  col_header_enum={}  use_min_max=off  min_val=-inf  max_val=inf  use_precision=off  precision=''  gain=1  offset=0  exp=1  use_mototune_group=off  mototune_group=motohawk_vardec_path(gcb)
  motohawk_calibration4 : MotoHawk_lib/Calibration & Probing Blocks/motohawk_calibration  nam='Li23MaxChargeTemp'  val=Li23MaxChargeTemp  storage=Calibration  show_more=off  name_source=Use Parameter  data_type=Inherit from 'Default Value'  read_level=1  write_level=1  ovr_cals=on  view_as=Number  enum_struct={'Disabled', 'Enabled'}  vector_style=Wide Row  use_help_units=off  help=''  units=''  use_header_enum=off  row_header_enum={}  col_header_enum={}  use_min_max=off  min_val=-inf  max_val=inf  use_precision=off  precision=''  gain=1  offset=0  exp=1  use_mototune_group=off  mototune_group=motohawk_vardec_path(gcb)
  motohawk_calibration5 : MotoHawk_lib/Calibration & Probing Blocks/motohawk_calibration  nam='Li23MinChargeTemp'  val=Li23MinChargeTemp  storage=Calibration  show_more=off  name_source=Use Parameter  data_type=Inherit from 'Default Value'  read_level=1  write_level=1  ovr_cals=on  view_as=Number  enum_struct={'Disabled', 'Enabled'}  vector_style=Wide Row  use_help_units=off  help=''  units=''  use_header_enum=off  row_header_enum={}  col_header_enum={}  use_min_max=off  min_val=-inf  max_val=inf  use_precision=off  precision=''  gain=1  offset=0  exp=1  use_mototune_group=off  mototune_group=motohawk_vardec_path(gcb)
  motohawk_calibration6 : MotoHawk_lib/Calibration & Probing Blocks/motohawk_calibration  nam='Li23MaxDischargeTemp'  val=Li23MaxDischargeTemp  storage=Calibration  show_more=off  name_source=Use Parameter  data_type=Inherit from 'Default Value'  read_level=1  write_level=1  ovr_cals=on  view_as=Number  enum_struct={'Disabled', 'Enabled'}  vector_style=Wide Row  use_help_units=off  help=''  units=''  use_header_enum=off  row_header_enum={}  col_header_enum={}  use_min_max=off  min_val=-inf  max_val=inf  use_precision=off  precision=''  gain=1  offset=0  exp=1  use_mototune_group=off  mototune_group=motohawk_vardec_path(gcb)
  motohawk_calibration7 : MotoHawk_lib/Calibration & Probing Blocks/motohawk_calibration  nam='Li23MinDischargeTemp'  val=Li23MinDischargeTemp  storage=Calibration  show_more=off  name_source=Use Parameter  data_type=Inherit from 'Default Value'  read_level=1  write_level=1  ovr_cals=on  view_as=Number  enum_struct={'Disabled', 'Enabled'}  vector_style=Wide Row  use_help_units=off  help=''  units=''  use_header_enum=off  row_header_enum={}  col_header_enum={}  use_min_max=off  min_val=-inf  max_val=inf  use_precision=off  precision=''  gain=1  offset=0  exp=1  use_mototune_group=off  mototune_group=motohawk_vardec_path(gcb)
  motohawk_calibration8 : MotoHawk_lib/Calibration & Probing Blocks/motohawk_calibration  nam='Li23MaxPackVoltage'  val=Li23MaxPackVoltage  storage=Calibration  show_more=off  name_source=Use Parameter  data_type=Inherit from 'Default Value'  read_level=1  write_level=1  ovr_cals=on  view_as=Number  enum_struct={'Disabled', 'Enabled'}  vector_style=Wide Row  use_help_units=off  help=''  units=''  use_header_enum=off  row_header_enum={}  col_header_enum={}  use_min_max=off  min_val=-inf  max_val=inf  use_precision=off  precision=''  gain=1  offset=0  exp=1  use_mototune_group=off  mototune_group=motohawk_vardec_path(gcb)
  motohawk_calibration9 : MotoHawk_lib/Calibration & Probing Blocks/motohawk_calibration  nam='Li23MinPackVoltage'  val=Li23MinPackVoltage  storage=Calibration  show_more=off  name_source=Use Parameter  data_type=Inherit from 'Default Value'  read_level=1  write_level=1  ovr_cals=on  view_as=Number  enum_struct={'Disabled', 'Enabled'}  vector_style=Wide Row  use_help_units=off  help=''  units=''  use_header_enum=off  row_header_enum={}  col_header_enum={}  use_min_max=off  min_val=-inf  max_val=inf  use_precision=off  precision=''  gain=1  offset=0  exp=1  use_mototune_group=off  mototune_group=motohawk_vardec_path(gcb)
  Li23Pack : Outport
  wires:
  motohawk_calibration/1 -> Mux/1  "MaxCellVoltage"
  motohawk_calibration1/1 -> Mux/2  "MinCellVoltage"
  motohawk_calibration2/1 -> Mux/3  "CurrentLimit"
  motohawk_calibration3/1 -> Mux/4  "RegenLimit"
  motohawk_calibration4/1 -> Mux/5  "MaxChargeTemp"
  motohawk_calibration5/1 -> Mux/6  "MinChargeTemp"
  motohawk_calibration6/1 -> Mux/7  "MaxDischargeTemp"
  motohawk_calibration7/1 -> Mux/8  "MinDischargeTemp"
  motohawk_calibration8/1 -> Mux/9  "MaxPackVoltage"
  motohawk_calibration9/1 -> Mux/10  "MinPackVoltage"
  motohawk_calibration10/1 -> Mux/11  "MotorCurrentScalar"
  motohawk_calibration11/1 -> Mux/12  "MotorRegenScalar"
  motohawk_calibration12/1 -> Mux/13  "MaxRegenVoltage"
  Mux/1 -> Li23Pack/1

== system GTA_PCMFirmware/Function/1 Inputs and Paramaters/Limits/Li7kWh ==
  Mux : Mux  Inputs=13
  motohawk_calibration : MotoHawk_lib/Calibration & Probing Blocks/motohawk_calibration  nam='Li7MaxCellVoltage'  val=Li7MaxCellVoltage  storage=Calibration  show_more=off  name_source=Use Parameter  data_type=Inherit from 'Default Value'  read_level=1  write_level=1  ovr_cals=on  view_as=Number  enum_struct={'Disabled', 'Enabled'}  vector_style=Wide Row  use_help_units=off  help=''  units=''  use_header_enum=off  row_header_enum={}  col_header_enum={}  use_min_max=off  min_val=-inf  max_val=inf  use_precision=off  precision=''  gain=1  offset=0  exp=1  use_mototune_group=off  mototune_group=motohawk_vardec_path(gcb)
  motohawk_calibration1 : MotoHawk_lib/Calibration & Probing Blocks/motohawk_calibration  nam='Li7MinCellVoltage'  val=Li7MinCellVoltage  storage=Calibration  show_more=off  name_source=Use Parameter  data_type=Inherit from 'Default Value'  read_level=1  write_level=1  ovr_cals=on  view_as=Number  enum_struct={'Disabled', 'Enabled'}  vector_style=Wide Row  use_help_units=off  help=''  units=''  use_header_enum=off  row_header_enum={}  col_header_enum={}  use_min_max=off  min_val=-inf  max_val=inf  use_precision=off  precision=''  gain=1  offset=0  exp=1  use_mototune_group=off  mototune_group=motohawk_vardec_path(gcb)
  motohawk_calibration10 : MotoHawk_lib/Calibration & Probing Blocks/motohawk_calibration  nam='Li7MotorCurrentScalar'  val=Li7MotorCurrentScalar  storage=Calibration  show_more=off  name_source=Use Parameter  data_type=Inherit from 'Default Value'  read_level=1  write_level=1  ovr_cals=on  view_as=Number  enum_struct={'Disabled', 'Enabled'}  vector_style=Wide Row  use_help_units=off  help=''  units=''  use_header_enum=off  row_header_enum={}  col_header_enum={}  use_min_max=off  min_val=-inf  max_val=inf  use_precision=off  precision=''  gain=1  offset=0  exp=1  use_mototune_group=off  mototune_group=motohawk_vardec_path(gcb)
  motohawk_calibration11 : MotoHawk_lib/Calibration & Probing Blocks/motohawk_calibration  nam='Li7MotorRegenScalar'  val=Li7MotorRegenScalar  storage=Calibration  show_more=off  name_source=Use Parameter  data_type=Inherit from 'Default Value'  read_level=1  write_level=1  ovr_cals=on  view_as=Number  enum_struct={'Disabled', 'Enabled'}  vector_style=Wide Row  use_help_units=off  help=''  units=''  use_header_enum=off  row_header_enum={}  col_header_enum={}  use_min_max=off  min_val=-inf  max_val=inf  use_precision=off  precision=''  gain=1  offset=0  exp=1  use_mototune_group=off  mototune_group=motohawk_vardec_path(gcb)
  motohawk_calibration12 : MotoHawk_lib/Calibration & Probing Blocks/motohawk_calibration  nam='Li7MaxRegenVoltage'  val=Li7MaxRegenVoltage  storage=Calibration  show_more=off  name_source=Use Parameter  data_type=Inherit from 'Default Value'  read_level=1  write_level=1  ovr_cals=on  view_as=Number  enum_struct={'Disabled', 'Enabled'}  vector_style=Wide Row  use_help_units=off  help=''  units=''  use_header_enum=off  row_header_enum={}  col_header_enum={}  use_min_max=off  min_val=-inf  max_val=inf  use_precision=off  precision=''  gain=1  offset=0  exp=1  use_mototune_group=off  mototune_group=motohawk_vardec_path(gcb)
  motohawk_calibration2 : MotoHawk_lib/Calibration & Probing Blocks/motohawk_calibration  nam='Li7CurrentLimit'  val=Li7CurrentLimit  storage=Calibration  show_more=off  name_source=Use Parameter  data_type=Inherit from 'Default Value'  read_level=1  write_level=1  ovr_cals=on  view_as=Number  enum_struct={'Disabled', 'Enabled'}  vector_style=Wide Row  use_help_units=off  help=''  units=''  use_header_enum=off  row_header_enum={}  col_header_enum={}  use_min_max=off  min_val=-inf  max_val=inf  use_precision=off  precision=''  gain=1  offset=0  exp=1  use_mototune_group=off  mototune_group=motohawk_vardec_path(gcb)
  motohawk_calibration3 : MotoHawk_lib/Calibration & Probing Blocks/motohawk_calibration  nam='Li7RegenLimit'  val=Li7RegenLimit  storage=Calibration  show_more=off  name_source=Use Parameter  data_type=Inherit from 'Default Value'  read_level=1  write_level=1  ovr_cals=on  view_as=Number  enum_struct={'Disabled', 'Enabled'}  vector_style=Wide Row  use_help_units=off  help=''  units=''  use_header_enum=off  row_header_enum={}  col_header_enum={}  use_min_max=off  min_val=-inf  max_val=inf  use_precision=off  precision=''  gain=1  offset=0  exp=1  use_mototune_group=off  mototune_group=motohawk_vardec_path(gcb)
  motohawk_calibration4 : MotoHawk_lib/Calibration & Probing Blocks/motohawk_calibration  nam='Li7MaxChargeTemp'  val=Li7MaxChargeTemp  storage=Calibration  show_more=off  name_source=Use Parameter  data_type=Inherit from 'Default Value'  read_level=1  write_level=1  ovr_cals=on  view_as=Number  enum_struct={'Disabled', 'Enabled'}  vector_style=Wide Row  use_help_units=off  help=''  units=''  use_header_enum=off  row_header_enum={}  col_header_enum={}  use_min_max=off  min_val=-inf  max_val=inf  use_precision=off  precision=''  gain=1  offset=0  exp=1  use_mototune_group=off  mototune_group=motohawk_vardec_path(gcb)
  motohawk_calibration5 : MotoHawk_lib/Calibration & Probing Blocks/motohawk_calibration  nam='Li7MinChargeTemp'  val=Li7MinChargeTemp  storage=Calibration  show_more=off  name_source=Use Parameter  data_type=Inherit from 'Default Value'  read_level=1  write_level=1  ovr_cals=on  view_as=Number  enum_struct={'Disabled', 'Enabled'}  vector_style=Wide Row  use_help_units=off  help=''  units=''  use_header_enum=off  row_header_enum={}  col_header_enum={}  use_min_max=off  min_val=-inf  max_val=inf  use_precision=off  precision=''  gain=1  offset=0  exp=1  use_mototune_group=off  mototune_group=motohawk_vardec_path(gcb)
  motohawk_calibration6 : MotoHawk_lib/Calibration & Probing Blocks/motohawk_calibration  nam='Li7MaxDischargeTemp'  val=Li7MaxDischargeTemp  storage=Calibration  show_more=off  name_source=Use Parameter  data_type=Inherit from 'Default Value'  read_level=1  write_level=1  ovr_cals=on  view_as=Number  enum_struct={'Disabled', 'Enabled'}  vector_style=Wide Row  use_help_units=off  help=''  units=''  use_header_enum=off  row_header_enum={}  col_header_enum={}  use_min_max=off  min_val=-inf  max_val=inf  use_precision=off  precision=''  gain=1  offset=0  exp=1  use_mototune_group=off  mototune_group=motohawk_vardec_path(gcb)
  motohawk_calibration7 : MotoHawk_lib/Calibration & Probing Blocks/motohawk_calibration  nam='Li7MinDischargeTemp'  val=Li7MinDischargeTemp  storage=Calibration  show_more=off  name_source=Use Parameter  data_type=Inherit from 'Default Value'  read_level=1  write_level=1  ovr_cals=on  view_as=Number  enum_struct={'Disabled', 'Enabled'}  vector_style=Wide Row  use_help_units=off  help=''  units=''  use_header_enum=off  row_header_enum={}  col_header_enum={}  use_min_max=off  min_val=-inf  max_val=inf  use_precision=off  precision=''  gain=1  offset=0  exp=1  use_mototune_group=off  mototune_group=motohawk_vardec_path(gcb)
  motohawk_calibration8 : MotoHawk_lib/Calibration & Probing Blocks/motohawk_calibration  nam='Li7MaxPackVoltage'  val=Li7MaxPackVoltage  storage=Calibration  show_more=off  name_source=Use Parameter  data_type=Inherit from 'Default Value'  read_level=1  write_level=1  ovr_cals=on  view_as=Number  enum_struct={'Disabled', 'Enabled'}  vector_style=Wide Row  use_help_units=off  help=''  units=''  use_header_enum=off  row_header_enum={}  col_header_enum={}  use_min_max=off  min_val=-inf  max_val=inf  use_precision=off  precision=''  gain=1  offset=0  exp=1  use_mototune_group=off  mototune_group=motohawk_vardec_path(gcb)
  motohawk_calibration9 : MotoHawk_lib/Calibration & Probing Blocks/motohawk_calibration  nam='Li7MinPackVoltage'  val=Li7MinPackVoltage  storage=Calibration  show_more=off  name_source=Use Parameter  data_type=Inherit from 'Default Value'  read_level=1  write_level=1  ovr_cals=on  view_as=Number  enum_struct={'Disabled', 'Enabled'}  vector_style=Wide Row  use_help_units=off  help=''  units=''  use_header_enum=off  row_header_enum={}  col_header_enum={}  use_min_max=off  min_val=-inf  max_val=inf  use_precision=off  precision=''  gain=1  offset=0  exp=1  use_mototune_group=off  mototune_group=motohawk_vardec_path(gcb)
  Li7Pack : Outport
  wires:
  motohawk_calibration/1 -> Mux/1  "MaxCellVoltage"
  motohawk_calibration1/1 -> Mux/2  "MinCellVoltage"
  motohawk_calibration2/1 -> Mux/3  "CurrentLimit"
  motohawk_calibration3/1 -> Mux/4  "RegenLimit"
  motohawk_calibration4/1 -> Mux/5  "MaxChargeTemp"
  motohawk_calibration5/1 -> Mux/6  "MinChargeTemp"
  motohawk_calibration6/1 -> Mux/7  "MaxDischargeTemp"
  motohawk_calibration7/1 -> Mux/8  "MinDischargeTemp"
  motohawk_calibration8/1 -> Mux/9  "MaxPackVoltage"
  motohawk_calibration9/1 -> Mux/10  "MinPackVoltage"
  motohawk_calibration10/1 -> Mux/11  "MotorCurrentScalar"
  motohawk_calibration11/1 -> Mux/12  "MotorRegenScalar"
  motohawk_calibration12/1 -> Mux/13  "MaxRegenVoltage"
  Mux/1 -> Li7Pack/1
